simulink model "LiftControl"  (R2020a)
settings: Solver=VariableStepAuto  StartTime=0.0  StopTime=100  RelTol=1e-3
settings Model: Creator=Admin  LastModifiedBy=Admin

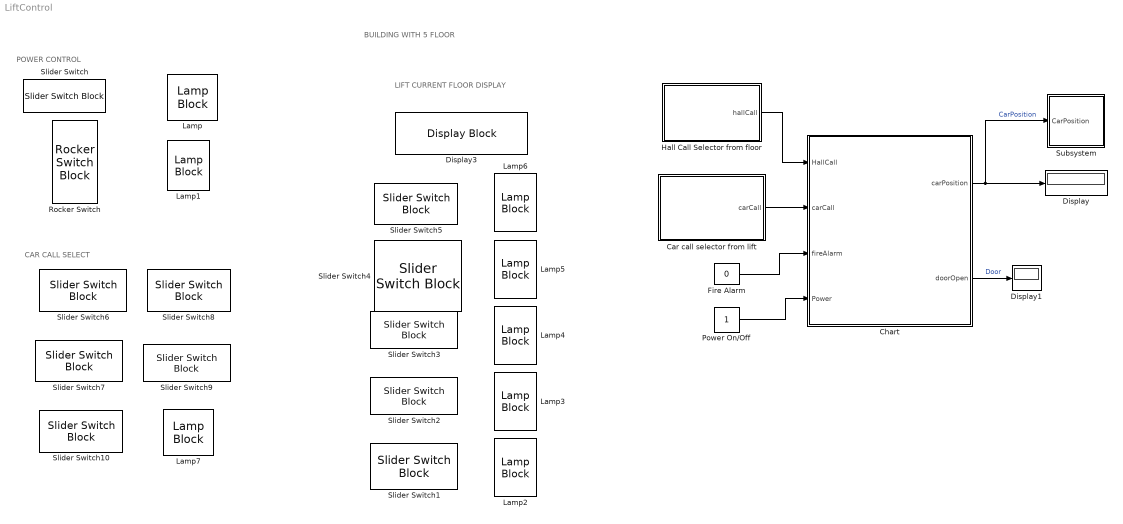
== system LiftControl ==
  note: BUILDING WITH 5 FLOOR
  note: LIFT CURRENT FLOOR DISPLAY
  note: CAR CALL SELECT
  note: POWER CONTROL
  Car call selector from lift : Subsystem
  Chart : Stateflow chart  TreatAsAtomicUnit=on
  Display : Display
  Display1 : Display
  Display3 : DisplayBlock  Format=short  Transparency=1
  Fire Alarm : Constant  Value=0
  Hall Call Selector from floor : Subsystem
  Lamp{,1..7} (8 alike) : LampBlock
  Power On/Off : Constant
  Rocker Switch : RockerSwitchBlock
      settings: Values={{'Off', 'On'}, [0 1]}
  Slider Switch{,1..10} (11 alike) : SliderSwitchBlock
      settings: Values={{'Off', 'On'}, [0 1]}
  Subsystem : Subsystem
  wires:
  Fire Alarm/1 -> Chart/3(fireAlarm)
  Power On/Off/1 -> Chart/4(Power)
  Chart/1(carPosition) -> Subsystem/1(CarPosition), Display/1  "CarPosition"
  Chart/2(doorOpen) -> Display1/1  "Door"
  Hall Call Selector from floor/1(hallCall) -> Chart/1(HallCall)
  Car call selector from lift/1(carCall) -> Chart/2(carCall)

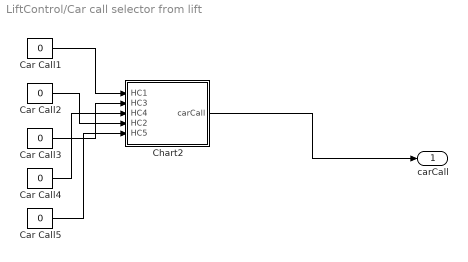
== system LiftControl/Car call selector from lift ==
  Car Call{1..5} (5 alike) : Constant  Value=0
  Chart2 : Stateflow chart  TreatAsAtomicUnit=on
  carCall : Outport
  wires:
  Car Call3/1 -> Chart2/2(HC3)
  Car Call1/1 -> Chart2/1(HC1)
  Car Call2/1 -> Chart2/4(HC2)
  Car Call4/1 -> Chart2/3(HC4)
  Car Call5/1 -> Chart2/5(HC5)
  Chart2/1(carCall) -> carCall/1

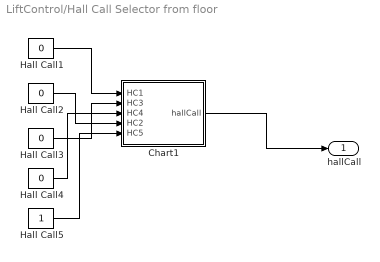
== system LiftControl/Hall Call Selector from floor ==
  Chart1 : Stateflow chart  TreatAsAtomicUnit=on
  Hall Call{1..4} (4 alike) : Constant  Value=0
  Hall Call5 : Constant
  hallCall : Outport
  wires:
  Hall Call2/1 -> Chart1/4(HC2)
  Hall Call1/1 -> Chart1/1(HC1)
  Chart1/1(hallCall) -> hallCall/1
  Hall Call4/1 -> Chart1/3(HC4)
  Hall Call3/1 -> Chart1/2(HC3)
  Hall Call5/1 -> Chart1/5(HC5)

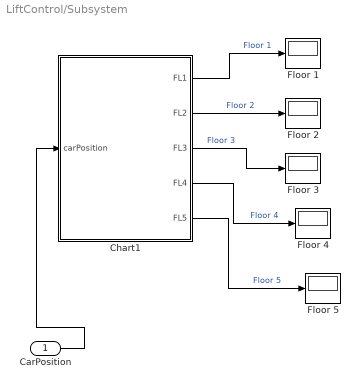
== system LiftControl/Subsystem ==
  CarPosition : Inport
  Chart1 : Stateflow chart  TreatAsAtomicUnit=on
  Floor {1..5} (5 alike) : Display
  wires:
  CarPosition/1 -> Chart1/1(carPosition)
  Chart1/1(FL1) -> Floor 1/1  "Floor 1"
  Chart1/2(FL2) -> Floor 2/1  "Floor 2"
  Chart1/4(FL4) -> Floor 4/1  "Floor 4"
  Chart1/3(FL3) -> Floor 3/1  "Floor 3"
  Chart1/5(FL5) -> Floor 5/1  "Floor 5"

== stateflow chart LiftControl/Hall Call Selector from floor/Chart1 ==
  (default) -> (junction 18) : % Hall call selector
  (junction 18) -> (junction 19) [order 1] : [HC1 > 0]
  (junction 18) -> (junction 20) [order 2]
  (junction 19) -> (junction 27) : {hallCall = 1;}
  (junction 20) -> (junction 21) [order 1] : [HC2 > 0]
  (junction 20) -> (junction 22) [order 2]
  (junction 21) -> (junction 26) : {hallCall = 2;}
  (junction 22) -> (junction 23) [order 1] : [HC3 > 0]
  (junction 22) -> (junction 32) [order 2]
  (junction 23) -> (junction 25) : {hallCall = 3;}
  (junction 32) -> (junction 34) [order 1] : [HC4 > 0]
  (junction 32) -> (junction 41) [order 2]
  (junction 34) -> (junction 36) : {hallCall = 4;}
  (junction 41) -> (junction 44) [order 1] : [HC5 > 0]
  (junction 41) -> (junction 24) [order 2] : {hallCall = 0;}
  (junction 44) -> (junction 39) : {hallCall = 5;}
  (junction 39) -> (junction 24)
  (junction 36) -> (junction 39)
  (junction 25) -> (junction 36)
  (junction 26) -> (junction 25)
  (junction 27) -> (junction 26)
  (junction 24) -> (junction 28)
  data: HC1 input; HC3 input; HC4 input; HC2 input; HC5 input; hallCall output

== stateflow chart LiftControl/Car call selector from lift/Chart2 ==
  (default) -> (junction 18) : % Hall call selector
  (junction 18) -> (junction 19) [order 1] : [HC1 > 0]
  (junction 18) -> (junction 20) [order 2]
  (junction 19) -> (junction 27) : {carCall = 1;}
  (junction 20) -> (junction 21) [order 1] : [HC2 > 0]
  (junction 20) -> (junction 22) [order 2]
  (junction 21) -> (junction 26) : {carCall = 2;}
  (junction 22) -> (junction 23) [order 1] : [HC3 > 0]
  (junction 22) -> (junction 32) [order 2]
  (junction 23) -> (junction 25) : {carCall = 3;}
  (junction 32) -> (junction 34) [order 1] : [HC4 > 0]
  (junction 32) -> (junction 41) [order 2]
  (junction 34) -> (junction 36) : {carCall = 4;}
  (junction 41) -> (junction 44) [order 1] : [HC5 > 0]
  (junction 41) -> (junction 24) [order 2] : {carCall = 0;}
  (junction 44) -> (junction 39) : {carCall = 5;}
  (junction 39) -> (junction 24)
  (junction 36) -> (junction 39)
  (junction 25) -> (junction 36)
  (junction 26) -> (junction 25)
  (junction 27) -> (junction 26)
  (junction 24) -> (junction 28)
  data: HC1 input; HC3 input; HC4 input; HC2 input; HC5 input; carCall output

== stateflow chart LiftControl/Chart ==
  state PowerControl [parallel]
    settings: executionOrder=1
    state Active
      state hallRequest
        en: callAccept = HallCall;
      state carRequest
        en: callAccept = carCall;
      (default) -> hallRequest
      carRequest -> carRequest [order 2] : arrive
      hallRequest -> carRequest : arrive
      carRequest -> hallRequest [order 1] : arrive[carCall == 0]
    state Idle
      doorOpen =1;
    (default) -> Idle : {carPosition =1;}
    Idle -> Active : [Power == 1]
    Active -> Idle : [Power == 0 || fireAlarm == 1]
  state Direction [parallel]
    settings: executionOrder=2
    state Up
      en: carPosition = carPosition +1;
    state Down
      en: carPosition = carPosition -1;
    state Start
      doorOpen =0;
    state Wait
      doorOpen =1;
    (default) -> Start
    Start -> Down [order 1] : [callAccept < carPosition]
    Start -> Up [order 2] : [callAccept > carPosition]
    Down -> Down [order 3]
    Wait -> Start : after(5,sec){doorOpen =0;}
    Down -> Wait [order 1] : [carPosition == callAccept]/{arrive}
    Down -> Wait [order 2] : [carPosition == HallCall || carPosition == carCall]
    Up -> Up [order 3]
    Up -> Wait [order 2] : [carPosition == HallCall || carPosition == carCall]
    Up -> Wait [order 1] : [carPosition == callAccept]/{arrive}
  (default) -> PowerControl
  data: HallCall input; carCall input; fireAlarm input; carPosition output; doorOpen output; Power input; callAccept local
  events: arrive local FUNCTION_CALL_EVENT

== stateflow chart LiftControl/Subsystem/Chart1 ==
  note: Do not put any code along
      | the transitions that run
      | down the right side!
  (default) -> (junction 26) : % Lift Display
      | {FL1=0;
      | FL2 = 0;
      | FL3 =0;
      | FL4 = 0;
      | FL5 =0;}
  (junction 26) -> (junction 27) [order 1] : [carPosition == 1]
  (junction 26) -> (junction 30) [order 2]
  (junction 27) -> (junction 28) : {FL1 =1;}
  (junction 28) -> (junction 29)
  (junction 29) -> (junction 33)
  (junction 30) -> (junction 31) [order 1] : [carPosition == 2]
  (junction 30) -> (junction 34) [order 2]
  (junction 31) -> (junction 32) : {FL2 = 1;}
  (junction 32) -> (junction 33)
  (junction 33) -> (junction 37)
  (junction 34) -> (junction 35) [order 1] : [carPosition == 3]
  (junction 34) -> (junction 38) [order 2]
  (junction 35) -> (junction 36) : {FL3 = 1;}
  (junction 36) -> (junction 37)
  (junction 37) -> (junction 41)
  (junction 38) -> (junction 39) [order 1] : [carPosition == 4]
  (junction 38) -> (junction 52) [order 2]
  (junction 39) -> (junction 40) : {FL4 = 1;}
  (junction 52) -> (junction 54) [order 1] : [carPosition == 5]
  (junction 40) -> (junction 41)
  (junction 52) -> (junction 42) [order 2]
  (junction 54) -> (junction 56) : {FL5 = 1;}
  (junction 41) -> (junction 58)
  (junction 56) -> (junction 58)
  (junction 58) -> (junction 43)
  (junction 43) -> (junction 42)
  (junction 42) -> (junction 44)
  data: carPosition input; FL1 output; FL2 output; FL3 output; FL4 output; FL5 output
